simulink library "PrerecordData"  (R2014a)
settings: Solver=ode45  SolverMode=SingleTasking  StartTime=0  StopTime=112.776  RelTol=1e-3
undefined symbols (not defined in the file): DataDescription
settings Model: Creator=Shad Laws  LastModifiedBy=cbeal

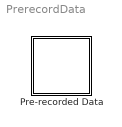
== system PrerecordData ==
  Pre-recorded Data : Subsystem  mask{filename='craig_2018-06-21_au.mat', timeflag=off, starttime=30, stoptime=80}
      mask prompts: filename "Name of data file to use"; timeflag "Customize start / stop times"; starttime "Start time"; stoptime "Stop time"
      mask init:
      | load(filename);
      | % get rid of xPC non-constant sample time
      | % anomoly... makes matching easier.
      | % round t to the nearest 0.0001 sec
      | t = round(t*10000)/10000;
      | 
      | if (~(exist('DataDescription')&exist('y')&exist('t')))
      | 	error('Invalid data file.');
      | end
      | 
      | % Truncate the y vector to get just the data described in DataDescription
      | y = y(:,1:sum([DataDescription.size]));
      | 
      | switch(timeflag);
      | 	case 'on';
      | 		set_param(gcs,'StopTime',num2str(stoptime));
      | 		set_param(gcs,'StartTime',num2str(starttime));
      | 	case 'off';
      | 		set_param(gcs,'StopTime',num2str(t(end)));
      | 		set_param(gcs,'StartTime',num2str(t(1)));
      | 	case 1;
      | 		set_param(gcs,'StopTime',num2str(stoptime));
      | 		set_param(gcs,'StartTime',num2str(starttime));
      | 	case 0;
      | 		set_param(gcs,'StopTime',num2str(t(end)));
      | 		set_param(gcs,'StartTime',num2str(t(1)));
      | end;
      mask Callback timeflag:
      | if (strcmp(get_param(gcb,'timeflag'),'off'))
      | 	set_param(gcb,'MaskEnables',{'on','on','off','off'});
      | else
      | 	set_param(gcb,'MaskEnables',{'on','on','on','on'});
      | end
      mask Display: disp('Data');

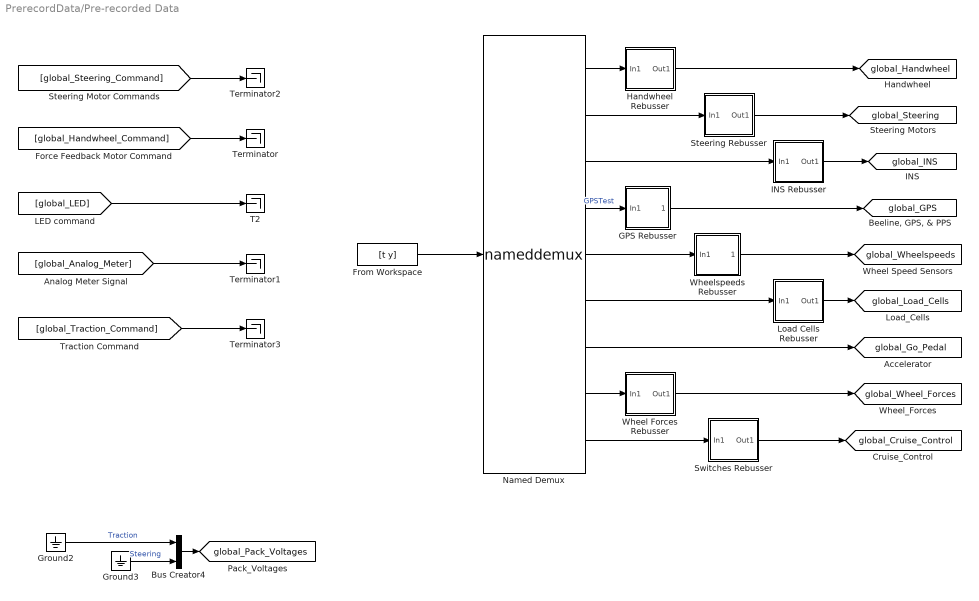
== system PrerecordData/Pre-recorded Data ==
  Bus Creator4 : BusCreator  Inputs=2
  From Workspace : FromWorkspace  VariableName=[t y]  SampleTime=0  OutputAfterFinalValue=Setting to zero
  GPS Rebusser : Subsystem
  Ground2 : Ground
  Ground3 : Ground
  Handwheel Rebusser : Subsystem
  INS Rebusser : Subsystem
  Load Cells Rebusser : Subsystem
  Named Demux : S-Function  FunctionName=nameddemux  Parameters=outputcount, outputsizes, outputindices, inputsize  EnableBusSupport=off  mask{desc=DataDescription, signals={'04 Handwheel' '01 Steering' '02 INS' '03 GPS' '06 Wheelspeeds' '10 Load Cells' '05 Accelerator' '15 Wheel Forces' '09 Switches' }}
      mask prompts: desc "Data description function name"; signals "Signal names"
      mask help:
      | Combines input signals into a single output vector, according to a structure that provides the names and sizes of each signal.
      |
      | The parameter below should be set to the name of a function which returns a 1xN structure array, where N is the number of input signals.  The structure should contain fields "size" which specifies the width of the input signal, and "name" which specifies its name.
      mask init:
      | outputcount=length(signals);
      | inputsize=sum([desc.size]);
      | 
      | indices=[1 cumsum([desc.size])+1];
      | 
      | if((outputcount<1)|(outputcount>50))
      | 	error('Inappropriate number of outputs.');
      | end
      | 
      | y=ones(1,outputcount);
      | 
      | for indx=1:outputcount,
      |     sig=signals{indx};
      | 	sigi=find(strcmp(sig,{desc.name}));
      |     if (length(sigi)==0)
      |         error(['Unable to find signal named "' sig '".']);
      |     end
      |     y(indx)=sigi;
      | end
      | 		
      | outputsizes=[desc(y).size];
      | outputindices=indices(y);
      | 
      | x=min(outputcount*ones(1,50),1:50);
      mask Display:
      | port_label('output',x(1),desc(y(x(1))).name);
      | port_label('output',x(2),desc(y(x(2))).name);
      | port_label('output',x(3),desc(y(x(3))).name);
      | port_label('output',x(4),desc(y(x(4))).name);
      | port_label('output',x(5),desc(y(x(5))).name);
      | port_label('output',x(6),desc(y(x(6))).name);
      | port_label('output',x(7),desc(y(x(7))).name);
      | port_label('output',x(8),desc(y(x(8))).name);
      | port_label('output',x(9),desc(y(x(9))).name);
      | port_label('output',x(10),desc(y(x(10))).name);
      | port_label('output',x(11),desc(y(x(11))).name);
      | port_label('output',x(12),desc(y(x(12))).name);
      | port_label('output',x(13),desc(y(x(13))).name);
      | port_label('output',x(14),desc(y(x(14))).name);
      | port_label('output',x(15),desc(y(x(15))).name);
      | port_label('output',x(16),desc(y(x(16))).name);
      | port_label('output',x(17),desc(y(x(17))).name);
      | port_label('output',x(18),desc(y(x(18))).name);
      | port_label('output',x(19),desc(y(x(19))).name);
      | port_label('output',x(20),desc(y(x(20))).name);
      | port_label('output',x(21),desc(y(x(21))).name);
      | port_label('output',x(22),desc(y(x(22))).name);
      | port_label('output',x(23),desc(y(x(23))).name);
      | port_label('output',x(24),desc(y(x(24))).name);
      | port_label('output',x(25),desc(y(x(25))).name);
      | port_label('output',x(26),desc(y(x(26))).name);
      | port_label('output',x(27),desc(y(x(27))).name);
      | port_label('output',x(28),desc(y(x(28))).name);
      | port_label('output',x(29),desc(y(x(29))).name);
      | port_label('output',x(30),desc(y(x(30))).name);
  Steering Rebusser : Subsystem
  Switches Rebusser : Subsystem
  T2 : Terminator
  Terminator{,1..3} (4 alike) : Terminator
  Wheel Forces Rebusser : Subsystem
  Wheelspeeds Rebusser : Subsystem
  tag scope: global_Cruise_Control=global, global_GPS=global, global_Go_Pedal=global, global_Handwheel=global, global_INS=global, global_Load_Cells=global, global_Pack_Voltages=global, global_Steering=global, global_Wheel_Forces=global, global_Wheelspeeds=global
  wires:
  Switches Rebusser/1(Out1) -> [global_Cruise_Control]
  Named Demux/9 -> Switches Rebusser/1(In1)
  Wheel Forces Rebusser/1(Out1) -> [global_Wheel_Forces]
  Named Demux/8 -> Wheel Forces Rebusser/1(In1)
  Named Demux/6 -> Load Cells Rebusser/1(In1)
  INS Rebusser/1(Out1) -> [global_INS]
  Bus Creator4/1 -> [global_Pack_Voltages]
  Ground3/1 -> Bus Creator4/2  "Steering"
  Ground2/1 -> Bus Creator4/1  "Traction"
  Named Demux/5 -> Wheelspeeds Rebusser/1(In1)
  Named Demux/2 -> Steering Rebusser/1(In1)
  Handwheel Rebusser/1(Out1) -> [global_Handwheel]
  Named Demux/1 -> Handwheel Rebusser/1(In1)
  [global_Traction_Command] -> Terminator3/1
  [global_Analog_Meter] -> Terminator1/1
  [global_Steering_Command] -> Terminator2/1
  [global_Handwheel_Command] -> Terminator/1
  Named Demux/3 -> INS Rebusser/1(In1)
  From Workspace/1 -> Named Demux/1
  [global_LED] -> T2/1
  Steering Rebusser/1(Out1) -> [global_Steering]
  GPS Rebusser/1(Out1) -> [global_GPS]
  Named Demux/4 -> GPS Rebusser/1(In1)  "GPSTest"
  Wheelspeeds Rebusser/1(Out1) -> [global_Wheelspeeds]
  Load Cells Rebusser/1(Out1) -> [global_Load_Cells]
  Named Demux/7 -> [global_Go_Pedal]

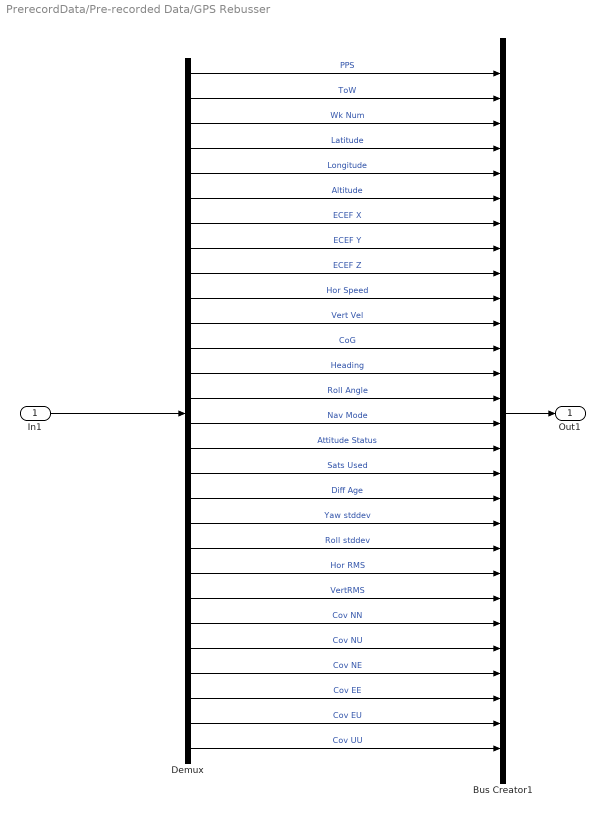
== system PrerecordData/Pre-recorded Data/GPS Rebusser ==
  In1 : Inport
  Bus Creator1 : BusCreator  Inputs=28
  Demux : Demux  Outputs=28
  Out1 : Outport
  wires:
  In1/1 -> Demux/1
  Demux/7 -> Bus Creator1/7  "ECEF X"
  Demux/4 -> Bus Creator1/4  "Latitude"
  Demux/5 -> Bus Creator1/5  "Longitude"
  Demux/6 -> Bus Creator1/6  "Altitude"
  Demux/3 -> Bus Creator1/3  "Wk Num"
  Demux/8 -> Bus Creator1/8  "ECEF Y"
  Demux/9 -> Bus Creator1/9  "ECEF Z"
  Demux/10 -> Bus Creator1/10  "Hor Speed"
  Demux/13 -> Bus Creator1/13  "Heading"
  Demux/11 -> Bus Creator1/11  "Vert Vel"
  Demux/12 -> Bus Creator1/12  "CoG"
  Demux/14 -> Bus Creator1/14  "Roll Angle"
  Demux/15 -> Bus Creator1/15  "Nav Mode"
  Demux/16 -> Bus Creator1/16  "Attitude Status"
  Demux/26 -> Bus Creator1/26  "Cov EE"
  Demux/27 -> Bus Creator1/27  "Cov EU"
  Demux/18 -> Bus Creator1/18  "Diff Age"
  Demux/19 -> Bus Creator1/19  "Yaw stddev"
  Demux/21 -> Bus Creator1/21  "Hor RMS"
  Demux/28 -> Bus Creator1/28  "Cov UU"
  Demux/17 -> Bus Creator1/17  "Sats Used"
  Demux/20 -> Bus Creator1/20  "Roll stddev"
  Demux/23 -> Bus Creator1/23  "Cov NN"
  Demux/22 -> Bus Creator1/22  "VertRMS"
  Demux/1 -> Bus Creator1/1  "PPS"
  Demux/2 -> Bus Creator1/2  "ToW"
  Bus Creator1/1 -> Out1/1
  Demux/24 -> Bus Creator1/24  "Cov NU"
  Demux/25 -> Bus Creator1/25  "Cov NE"

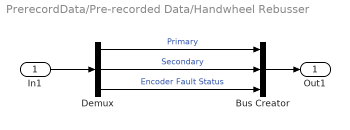
== system PrerecordData/Pre-recorded Data/Handwheel Rebusser ==
  In1 : Inport
  Bus Creator : BusCreator  Inputs=3
  Demux : Demux  Outputs=3
  Out1 : Outport
  wires:
  Bus Creator/1 -> Out1/1
  In1/1 -> Demux/1
  Demux/3 -> Bus Creator/3  "Encoder Fault Status"
  Demux/1 -> Bus Creator/1  "Primary"
  Demux/2 -> Bus Creator/2  "Secondary"

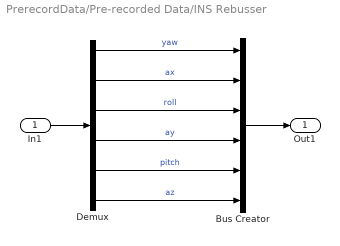
== system PrerecordData/Pre-recorded Data/INS Rebusser ==
  In1 : Inport
  Bus Creator : BusCreator  Inputs=6
  Demux : Demux  Outputs=6
  Out1 : Outport
  wires:
  Bus Creator/1 -> Out1/1
  In1/1 -> Demux/1
  Demux/4 -> Bus Creator/4  "ay"
  Demux/5 -> Bus Creator/5  "pitch"
  Demux/6 -> Bus Creator/6  "az"
  Demux/1 -> Bus Creator/1  "yaw"
  Demux/2 -> Bus Creator/2  "ax"
  Demux/3 -> Bus Creator/3  "roll"

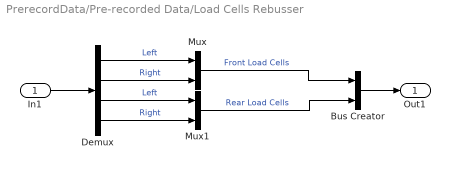
== system PrerecordData/Pre-recorded Data/Load Cells Rebusser ==
  In1 : Inport
  Bus Creator : BusCreator  Inputs=2
  Demux : Demux
  Mux : Mux  Inputs=2
  Mux1 : Mux  Inputs=2
  Out1 : Outport
  wires:
  Demux/2 -> Mux/2  "Right"
  Demux/1 -> Mux/1  "Left"
  Demux/4 -> Mux1/2  "Right"
  Demux/3 -> Mux1/1  "Left"
  Mux/1 -> Bus Creator/1  "Front Load Cells"
  Mux1/1 -> Bus Creator/2  "Rear Load Cells"
  In1/1 -> Demux/1
  Bus Creator/1 -> Out1/1

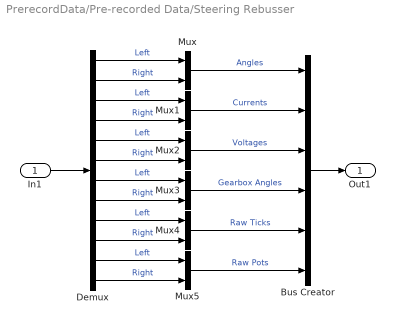
== system PrerecordData/Pre-recorded Data/Steering Rebusser ==
  In1 : Inport
  Bus Creator : BusCreator  Inputs=6
  Demux : Demux  Outputs=12
  Mux{,1..5} (6 alike) : Mux  Inputs=2
  Out1 : Outport
  wires:
  Bus Creator/1 -> Out1/1
  In1/1 -> Demux/1
  Mux/1 -> Bus Creator/1  "Angles"
  Mux1/1 -> Bus Creator/2  "Currents"
  Mux2/1 -> Bus Creator/3  "Voltages"
  Mux3/1 -> Bus Creator/4  "Gearbox Angles"
  Mux4/1 -> Bus Creator/5  "Raw Ticks"
  Mux5/1 -> Bus Creator/6  "Raw Pots"
  Demux/1 -> Mux/1  "Left"
  Demux/2 -> Mux/2  "Right"
  Demux/4 -> Mux1/2  "Right"
  Demux/3 -> Mux1/1  "Left"
  Demux/6 -> Mux2/2  "Right"
  Demux/5 -> Mux2/1  "Left"
  Demux/7 -> Mux3/1  "Left"
  Demux/8 -> Mux3/2  "Right"
  Demux/9 -> Mux4/1  "Left"
  Demux/10 -> Mux4/2  "Right"
  Demux/11 -> Mux5/1  "Left"
  Demux/12 -> Mux5/2  "Right"

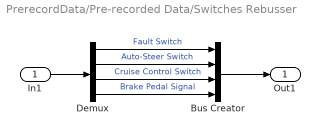
== system PrerecordData/Pre-recorded Data/Switches Rebusser ==
  In1 : Inport
  Bus Creator : BusCreator
  Demux : Demux
  Out1 : Outport
  wires:
  Bus Creator/1 -> Out1/1
  In1/1 -> Demux/1
  Demux/1 -> Bus Creator/1  "Fault Switch"
  Demux/2 -> Bus Creator/2  "Auto-Steer Switch"
  Demux/3 -> Bus Creator/3  "Cruise Control Switch"
  Demux/4 -> Bus Creator/4  "Brake Pedal Signal"

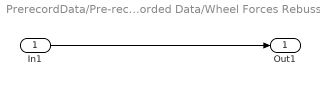
== system PrerecordData/Pre-recorded Data/Wheel Forces Rebusser ==
  In1 : Inport
  Out1 : Outport
  wires:
  In1/1 -> Out1/1

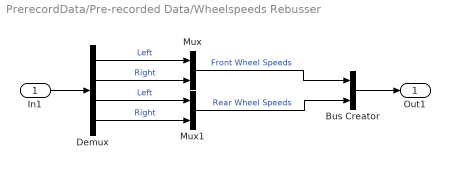
== system PrerecordData/Pre-recorded Data/Wheelspeeds Rebusser ==
  In1 : Inport
  Bus Creator : BusCreator  Inputs=2
  Demux : Demux
  Mux : Mux  Inputs=2
  Mux1 : Mux  Inputs=2
  Out1 : Outport
  wires:
  In1/1 -> Demux/1
  Demux/2 -> Mux/2  "Right"
  Demux/1 -> Mux/1  "Left"
  Demux/4 -> Mux1/2  "Right"
  Demux/3 -> Mux1/1  "Left"
  Bus Creator/1 -> Out1/1
  Mux/1 -> Bus Creator/1  "Front Wheel Speeds"
  Mux1/1 -> Bus Creator/2  "Rear Wheel Speeds"
